simulink model "H637"  (Simulink 7.3)
settings: Solver=ode45  StartTime=0.0  StopTime=10  RelTol=1e-4
libraries: simulink x1
settings Model: Creator=Admin  LastModifiedBy=Sainquake
settings DebuggingCC: StrictBusMsg=ErrorLevel1

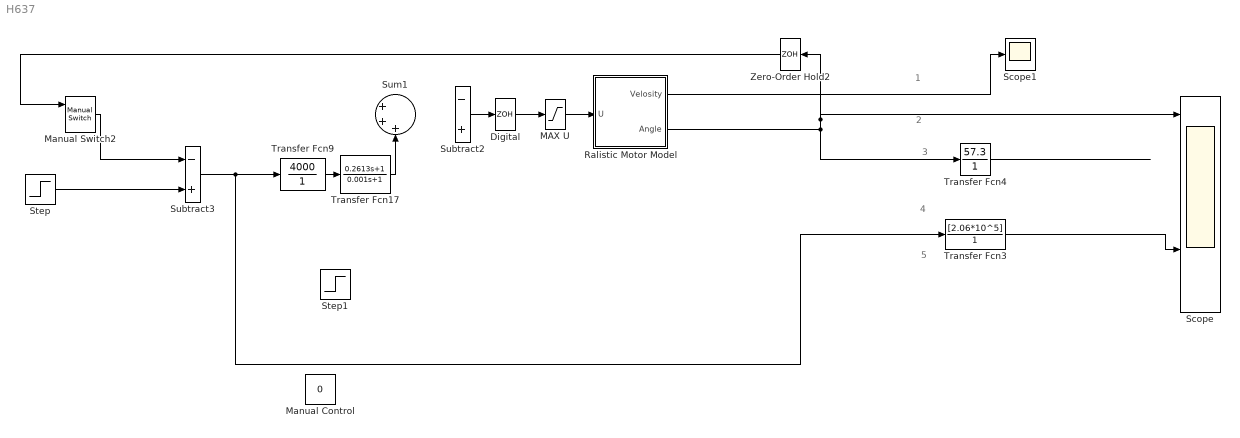
== system H637 ==
  note: 1
  note: 2
  note: 3
  note: 4
  note: 5
  Digital : ZeroOrderHold  SampleTime=1/19531.25
  MAX U : Saturate  UpperLimit=27  LowerLimit=-27
  Manual Control : Constant  Value=0
  Manual Switch2 : simulink/Signal Routing/Manual Switch  SystemSampleTime=-1  sw=1  action=0  varsize=off
  Ralistic Motor Model : Subsystem  TreatAsAtomicUnit=on
  Scope : Scope  NumInputPorts=5
      settings: TimeRange=1  YMin=0.83~-1~-1~26000~-1  YMax=0.875~1~1~35000~1  MaxDataPoints=5000000
  Scope1 : Scope
      settings: MaxDataPoints=500000
  Step : Step  Time=0.5  SampleTime=0
  Step1 : Step  Time=5  After=20  SampleTime=0
  Subtract2 : Sum  Inputs=-+
  Subtract3 : Sum  Inputs=-+
  Sum1 : Sum  Inputs=|+++
  Transfer Fcn17 : TransferFcn  Numerator=[0.2613 1]  Denominator=[0.001 1]
  Transfer Fcn3 : TransferFcn  Numerator=[2.06*10^5]  Denominator=[ 1 ]
  Transfer Fcn4 : TransferFcn  Numerator=[57.3]  Denominator=[ 1 ]
  Transfer Fcn9 : TransferFcn  Numerator=4000  Denominator=[ 1 ]
  Zero-Order Hold2 : ZeroOrderHold  SampleTime=1/25000
  wires:
  Ralistic Motor Model/2(Angle) -> Transfer Fcn4/1, Zero-Order Hold2/1, Scope/1
  Subtract3/1 -> Transfer Fcn3/1, Transfer Fcn9/1
  Transfer Fcn9/1 -> Transfer Fcn17/1
  Manual Switch2/1 -> Subtract3/1
  Transfer Fcn4/1 -> ?
  Transfer Fcn3/1 -> Scope/4
  Zero-Order Hold2/1 -> Manual Switch2/1
  MAX U/1 -> Ralistic Motor Model/1(U)
  Digital/1 -> MAX U/1
  Step/1 -> Subtract3/2
  Transfer Fcn17/1 -> Sum1/3
  Subtract2/1 -> Digital/1
  Ralistic Motor Model/1(Velosity) -> Scope1/1

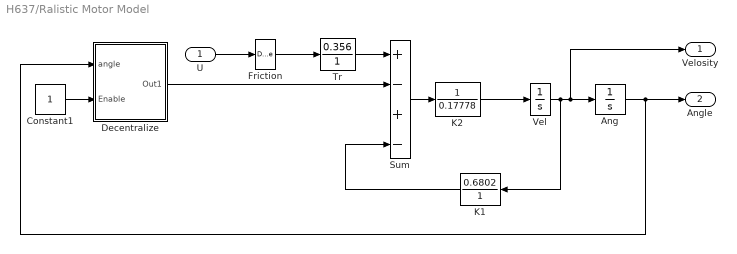
== system H637/Ralistic Motor Model ==
  U : Inport  OutDataType=fixdt(1, 16)  OutScaling=2^0
  Ang : Integrator
  Constant1 : Constant  OutDataType=fixdt(1, 16)  OutScaling=2^0
  Decentralize : Subsystem  TreatAsAtomicUnit=on
  Friction : DeadZone  LowerValue=-1.4  UpperValue=1.4  SaturateOnIntegerOverflow=on
  K1 : TransferFcn  Numerator=[0.6802]  Denominator=[ 1]
  K2 : TransferFcn  Denominator=0.17778
  Sum : Sum  Inputs=+-+-
  Tr : TransferFcn  Numerator=[0.356]  Denominator=[ 1 ]
  Vel : Integrator
  Velosity : Outport  OutDataType=fixdt(1, 16)  OutScaling=2^0
  Angle : Outport  Port=2  OutDataType=fixdt(1, 16)  OutScaling=2^0
  wires:
  Sum/1 -> K2/1
  K2/1 -> Vel/1
  Ang/1 -> Decentralize/1(angle), Angle/1
  K1/1 -> Sum/4
  Tr/1 -> Sum/1
  Decentralize/1(Out1) -> Sum/2
  Friction/1 -> Tr/1
  U/1 -> Friction/1
  Constant1/1 -> Decentralize/2(Enable)
  Vel/1 -> K1/1, Ang/1, Velosity/1

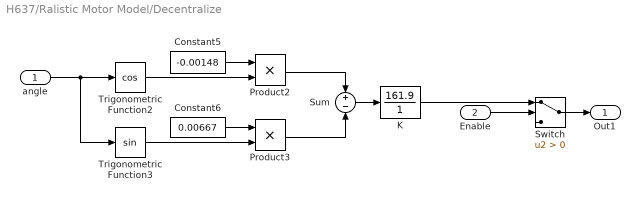
== system H637/Ralistic Motor Model/Decentralize ==
  angle : Inport  OutDataType=fixdt(1, 16)  OutScaling=2^0
  Enable : Inport  Port=2  OutDataType=fixdt(1, 16)  OutScaling=2^0
  Constant5 : Constant  Value=-0.00148
  Constant6 : Constant  Value=0.00667
  K : TransferFcn  Numerator=[161.9]  Denominator=[ 1 ]
  Product2 : Product  RndMeth=Zero
  Product3 : Product  RndMeth=Zero
  Sum : Sum  Inputs=+|-  OutDataType=fixdt(1, 16)  OutScaling=2^0
  Switch : Switch  Criteria=u2 > Threshold  OutDataType=fixdt(1, 16)  OutScaling=2^0
  Trigonometric Function2 : Trigonometry  Operator=cos
  Trigonometric Function3 : Trigonometry
  Out1 : Outport  OutDataType=fixdt(1, 16)  OutScaling=2^0
  wires:
  Constant5/1 -> Product2/1
  Trigonometric Function2/1 -> Product2/2
  Constant6/1 -> Product3/1
  Trigonometric Function3/1 -> Product3/2
  Product3/1 -> Sum/2
  Product2/1 -> Sum/1
  Sum/1 -> K/1
  K/1 -> Switch/1
  angle/1 -> Trigonometric Function2/1, Trigonometric Function3/1
  Enable/1 -> Switch/2
  Switch/1 -> Out1/1
